simulink model "exakt_mimo"  (Simulink 2.20)
settings: Solver=ode45  StartTime=0.0  StopTime=5.0  MaxStep=0.1  RelTol=1e-3  AbsTol=1e-6
libraries: NelinSys x4
CloseFcn:
  | ;slview('closediagram',bdroot);
settings Model: ConsistencyChecking=off  RTWPlaceOutputsASAP=off

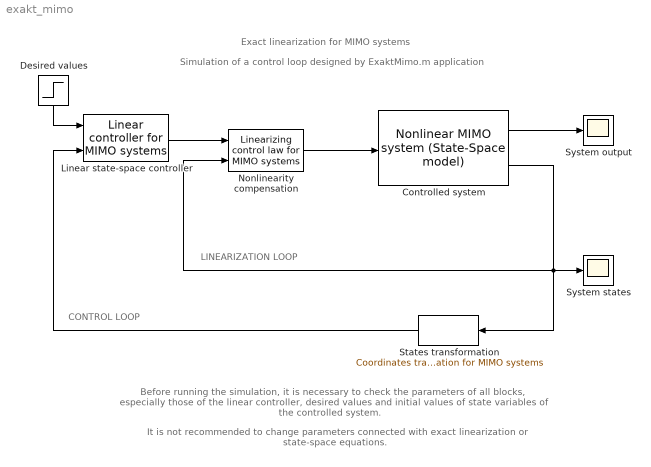
== system exakt_mimo ==
  note: LINEARIZATION LOOP
  note: CONTROL LOOP
  note: Exact linearization for MIMO systems
  note: Simulation of a control loop designed by ExaktMimo.m application
  note: Before running the simulation, it is necessary to check the parameters of all blocks, especially those
      | of the linear controller, desired values and initial values of state variables of the controlled system.
  note: It is not recommended to change parameters connected with exact linearization or state-space equations.
  " Desired values" : Step  Orientation=down  Time=[1 0]  Before=[0 0]  After=[2800/9.55 0.26]
  Controlled system : NelinSys/Nonlinear Systems Synthesis/Nonlinear MIMO system (State-Space model)  n=n  Fp=F  Gp=G  Hp=H  pp=[0; 0; 1e-9]
  Linear state-space controller : NelinSys/Nonlinear Systems Synthesis/Exact Linearization Blocks/Linear controller for MIMO systems  r=r  nout=nout  kor=[-20 -20 -20]  integ=off
  Nonlinearity compensation : NelinSys/Nonlinear Systems Synthesis/Exact Linearization Blocks/Linearizing control law for MIMO systems  n=n  nout=nout  vzorecP=u
  States transformation : NelinSys/Nonlinear Systems Synthesis/Exact Linearization Blocks/Coordinates transformation for MIMO systems  Orientation=left  n=n  r=r  Zp=qx
  System output : Scope
      settings: TickLabels=on  TimeRange=auto  YMin=-5  YMax=5  SaveToWorkspace=off  SaveName=ScopeData
  System states : Scope
      settings: TickLabels=on  TimeRange=auto  YMin=-5  YMax=5  SaveToWorkspace=off  SaveName=ScopeData
  wires:
  Linear state-space controller/1 -> Nonlinearity compensation/1
  States transformation/1 -> Linear state-space controller/2
  " Desired values"/1 -> Linear state-space controller/1
  Controlled system/2 -> States transformation/1, Nonlinearity compensation/2, System states/1
  Controlled system/1 -> System output/1
  Nonlinearity compensation/1 -> Controlled system/1
